simulink model "Appl_HeatFault_CtrlModel"  (R2018b)
settings: configuration reference "CodeConfig_10_ms" (kept outside this file)
undefined symbols (not defined in the file): CAL_CmdOpenTime, CAL_CmdShortTime, CAL_NTCOpenTime, CAL_NTCOverTime, CAL_NTCShortTime, CAL_NTCWaitTime, D_HEATFALUT_CmdOpenLoad, D_HEATFALUT_CmdOpenLoad_W, D_HEATFALUT_CmdShortToGnd, D_HEATFALUT_NtcMax, D_HEATFALUT_NtcMin, D_HEATFALUT_NtcOpenLoad, D_HEATFALUT_NtcShortToGnd, FALSE, TRUE
libraries: DareLib x32, simulink x1
(part 2 of 2)

== stateflow chart Appl_HeatFault_CtrlModel/LogicCtrl/HeatDiagnoseCtrl/HeatDiagnoseDeal/HeatCmdDiagnoseFunction2/HeatCmdDiagnose ==
  state HeatCmdDiagnosis
    state CmdShortToGND
      ex:
      ShortTimer = 0;
      (default) -> (junction 25)
      CmdShortToGND -> (junction 25) [order 1]
      (junction 25) -> (junction 28) [order 1] : /* 未超时 */
          | [CAL_CmdShortTime > ShortTimer]
      (junction 25) -> (junction 30) [order 2] : {ShortTimer = CAL_CmdShortTime;
          | HeatCmdFault = enHeatCmdFault.EN_HEAT_FAULT_GND;
          | HeatCmdFault4DTC = enHeatCmdFault.EN_HEAT_FAULT_GND;}
      (junction 28) -> (junction 32) : {ShortTimer++;}
      (junction 32) -> (junction 30)
      (junction 30) -> (junction 35)
    state ShortLow
    state Default
      en:
      OpenTimer = 0;
      ShortTimer = 0;
      HeatCmdFault =  enHeatCmdFault.EN_HEAT_FAULT_NONE;
      RecoverTimer = 0;
      (default) -> (junction 80)
      Default -> (junction 80) [order 1]
      (junction 80) -> (junction 83) [order 1] : /* 未超时 */
          | [CAL_CmdShortTime > RecoverTimer]
      (junction 80) -> (junction 89) [order 2] : {RecoverTimer = CAL_CmdShortTime;
          | HeatCmdFault4DTC =  enHeatCmdFault.EN_HEAT_FAULT_NONE;}
      (junction 83) -> (junction 84) : {RecoverTimer++;}
      (junction 84) -> (junction 89)
      (junction 89) -> (junction 91)
    state CmdOpenLoad
      ex:
      OpenTimer = 0;
      (default) -> (junction 46)
      CmdOpenLoad -> (junction 46) [order 1]
      (junction 46) -> (junction 43) [order 1] : /* 未超时 */
          | [CAL_CmdOpenTime > OpenTimer]
      (junction 46) -> (junction 47) [order 2] : {OpenTimer = CAL_CmdOpenTime;
          | HeatCmdFault = enHeatCmdFault.EN_HEAT_FAULT_OPEN;
          | HeatCmdFault4DTC = enHeatCmdFault.EN_HEAT_FAULT_OPEN;}
      (junction 43) -> (junction 48) : {OpenTimer++;}
      (junction 48) -> (junction 47)
      (junction 47) -> (junction 40)
    state OpenLow
    CmdShortToGND -> ShortLow [order 1] : /* 低电平 */
        | [enHeatIoSts.EN_HEAT_IO_LOW == HeatIOSts]
    ShortLow -> CmdShortToGND : /* 高电平 */
        | [enHeatIoSts.EN_HEAT_IO_HIGH == HeatIOSts]
    (junction 76) -> CmdShortToGND [order 1] : [FaultType == enHeatCmdFault.EN_HEAT_FAULT_GND]
    Default -> CmdShortToGND [order 1] : /* 输出电流对地短路 */
        | [D_HEATFALUT_CmdShortToGnd < HeatIS]
    CmdShortToGND -> Default [order 2] : /* 输出电流对地短路恢复 */
        | [D_HEATFALUT_CmdShortToGnd >= HeatIS]
    CmdOpenLoad -> CmdShortToGND [order 3] : /* 输出电流对地短路 */
        | [D_HEATFALUT_CmdShortToGnd < HeatIS]
    CmdShortToGND -> CmdOpenLoad [order 3] : /* 输出电流开路 */
        | [D_HEATFALUT_CmdOpenLoad_W > HeatIS]
    (default) -> (junction 76)
    (junction 76) -> Default [order 3]
    (junction 76) -> CmdOpenLoad [order 2] : [FaultType == enHeatCmdFault.EN_HEAT_FAULT_OPEN]
    Default -> CmdOpenLoad [order 2] : /* 输出电流开路 */
        | [D_HEATFALUT_CmdOpenLoad_W > HeatIS]
    CmdOpenLoad -> Default [order 2] : /* 输出电流开路恢复 */
        | [D_HEATFALUT_CmdOpenLoad_W <= HeatIS]
    CmdOpenLoad -> OpenLow [order 1] : /* 低电平 */
        | [enHeatIoSts.EN_HEAT_IO_LOW == HeatIOSts]
    OpenLow -> CmdOpenLoad : /* 高电平 */
        | [enHeatIoSts.EN_HEAT_IO_HIGH == HeatIOSts]
  state HeatCmdClose
    en:
    OpenTimer = 0;
    ShortTimer = 0;
    HeatCmdFault = enHeatCmdFault.EN_HEAT_FAULT_NONE;
    ex:
    HeatCmdFault4DTC = FaultType;
  (default) -> HeatCmdClose
  HeatCmdClose -> HeatCmdDiagnosis : /* 加热CMD */
      | [TRUE == HeatCmd]
  HeatCmdDiagnosis -> HeatCmdClose : /* 无加热CMD */
      | [TRUE != HeatCmd]
  data: HeatIOSts input Enum: enHeatIoSts; HeatCmd input uint8; HeatIS input uint16; HeatCmdFault output Enum: enHeatCmdFault; ShortTimer local uint8; OpenTimer local uint8; CAL_CmdShortTime parameter; CAL_CmdOpenTime parameter; D_HEATFALUT_CmdShortToGnd parameter; D_HEATFALUT_CmdOpenLoad_W parameter; TRUE parameter; HeatCmdFault4DTC output Enum: enHeatCmdFault; FaultType input; RecoverTimer local uint8

== stateflow chart Appl_HeatFault_CtrlModel/LogicCtrl/HeatDiagnoseCtrl/HeatDiagnoseDeal/HeatNTCDiagnoseFunction1/HeatCmdDiagnose ==
  state NTCShortToGND
    ex:
    ShortTimer = 0;
    (default) -> (junction 77)
    NTCShortToGND -> (junction 77) [order 1]
    (junction 77) -> (junction 80) [order 1] : /* 短地超时 */
        | [CAL_NTCShortTime > ShortTimer]
    (junction 77) -> (junction 82) [order 2] : {ShortTimer = CAL_NTCShortTime;
        | HeatNTCFault = enHeatNtcFault.EN_NTC_FAULT_GND;}
    (junction 80) -> (junction 84) : {ShortTimer++;}
    (junction 84) -> (junction 82)
    (junction 82) -> (junction 87)
  state Default
    en:
    WaitAquireTimer = 1;
    RecoveryTimer = 0;
    ex:
    WaitAquireTimer = 0;
    (default) -> (junction 64)
    (junction 64) -> (junction 69) [order 1] : /* 等待超时 */
        | [CAL_NTCWaitTime  > WaitAquireTimer]
    Default -> (junction 64) [order 1]
    (junction 69) -> (junction 71) : {WaitAquireTimer ++;}
    (junction 64) -> (junction 67) [order 2] : {WaitAquireTimer = CAL_NTCWaitTime;}
    (junction 71) -> (junction 67)
    (junction 67) -> (junction 74)
    (junction 74) -> (junction 139) [order 1] : [HeatNTCFault != enHeatNtcFault.EN_NTC_FAULT_NONE]
    (junction 74) -> (junction 162) [order 2]
    (junction 139) -> (junction 141) : {RecoveryTimer++; }
    (junction 141) -> (junction 143) [order 1] : /* NTC不可信故障*/
        | [HeatNTCFault == enHeatNtcFault.EN_NTC_FAULT_UNC]
    (junction 143) -> (junction 145) [order 1] : [/*计时超过5s*/
        | CAL_NTCOverTime < RecoveryTimer]
    (junction 141) -> (junction 152) [order 2]
    (junction 143) -> (junction 158) [order 2]
    (junction 145) -> (junction 150) : {RecoveryTimer = CAL_NTCOverTime;
        | HeatNTCFault = enHeatNtcFault.EN_NTC_FAULT_NONE;}
    (junction 152) -> (junction 154) [order 1] : [/*开路和短地时间皆为1s*/
        | CAL_NTCOpenTime < RecoveryTimer]
    (junction 152) -> (junction 160) [order 2]
    (junction 154) -> (junction 156) : {RecoveryTimer = CAL_NTCOpenTime;
        | HeatNTCFault = enHeatNtcFault.EN_NTC_FAULT_NONE;}
    (junction 162) -> (junction 160)
    (junction 156) -> (junction 160)
    (junction 158) -> (junction 156)
    (junction 150) -> (junction 158)
    (junction 160) -> (junction 168)
  state NTCOpenLoad
    ex:
    OpenTimer = 0;
    (default) -> (junction 94)
    NTCOpenLoad -> (junction 94) [order 1]
    (junction 94) -> (junction 92) [order 1] : /* 开路超时 */
        | [CAL_NTCOpenTime  > OpenTimer]
    (junction 94) -> (junction 95) [order 2] : {OpenTimer = CAL_NTCOpenTime;
        | HeatNTCFault = enHeatNtcFault.EN_NTC_FAULT_OPEN;}
    (junction 92) -> (junction 97) : {OpenTimer ++;}
    (junction 97) -> (junction 95)
    (junction 95) -> (junction 100)
  state NTCOverRange
    ex:
    OverTimer = 0;
    (default) -> (junction 105)
    NTCOverRange -> (junction 105) [order 1]
    (junction 105) -> (junction 108) [order 1] : /* 不可信超时 */
        | [CAL_NTCOverTime   > OverTimer]
    (junction 105) -> (junction 109) [order 2] : {OverTimer = CAL_NTCOverTime ;
        | HeatNTCFault = enHeatNtcFault.EN_NTC_FAULT_UNC;}
    (junction 108) -> (junction 110) : {OverTimer ++;}
    (junction 110) -> (junction 109)
    (junction 109) -> (junction 112)
  NTCShortToGND -> Default [order 1] : /* 对地短路 */
      | [D_HEATFALUT_NtcShortToGnd < HeatNTC]
  Default -> NTCShortToGND [order 1] : /* 对地恢复 */
      | [D_HEATFALUT_NtcShortToGnd >= HeatNTC ...
      | && CAL_NTCWaitTime <= WaitAquireTimer]
  (default) -> Default
  Default -> NTCOpenLoad [order 2] : /* NTC开路 */
      | [D_HEATFALUT_NtcOpenLoad < HeatNTC ...
      | && CAL_NTCWaitTime <= WaitAquireTimer]
  NTCOpenLoad -> Default [order 1] : /* NTC开路恢复*/
      | [D_HEATFALUT_NtcOpenLoad >= HeatNTC]
  Default -> NTCOverRange [order 3] : /* NTC 不可信 */
      | [(NtcMax < HeatNTC ...
      | || NtcMin > HeatNTC) ...
      | && CAL_NTCWaitTime <= WaitAquireTimer]
  NTCOverRange -> Default [order 1] : /* NTC不可信恢复 */
      | [(NtcMax >= HeatNTC && NtcMin <= HeatNTC) ...
      | || D_HEATFALUT_NtcOpenLoad < HeatNTC ...
      | || D_HEATFALUT_NtcShortToGnd >= HeatNTC]
  data: HeatNTC input uint16; HeatNTCFault output Enum: enHeatNtcFault; ShortTimer local uint16; WaitAquireTimer local uint16; OpenTimer local uint16; OverTimer local uint16; CAL_NTCOpenTime parameter; CAL_NTCOverTime parameter; CAL_NTCShortTime parameter; CAL_NTCWaitTime parameter; D_HEATFALUT_NtcOpenLoad parameter; D_HEATFALUT_NtcShortToGnd parameter; RecoveryTimer local uint16; NtcMin input uint16; NtcMax input uint16

== stateflow chart Appl_HeatFault_CtrlModel/LogicCtrl/HeatDiagnoseCtrl/HeatDiagnoseDeal/HeatNTCDiagnoseFunction2/HeatCmdDiagnose ==
  state NTCShortToGND
    ex:
    ShortTimer = 0;
    (default) -> (junction 77)
    NTCShortToGND -> (junction 77) [order 1]
    (junction 77) -> (junction 80) [order 1] : /* 短地超时 */
        | [CAL_NTCShortTime > ShortTimer]
    (junction 77) -> (junction 82) [order 2] : {ShortTimer = CAL_NTCShortTime;
        | HeatNTCFault = enHeatNtcFault.EN_NTC_FAULT_GND;}
    (junction 80) -> (junction 84) : {ShortTimer++;}
    (junction 84) -> (junction 82)
    (junction 82) -> (junction 87)
  state Default
    en:
    WaitAquireTimer = 1;
    RecoveryTimer = 0;
    ex:
    WaitAquireTimer = 0;
    (default) -> (junction 64)
    (junction 64) -> (junction 69) [order 1] : /* 等待超时 */
        | [CAL_NTCWaitTime  > WaitAquireTimer]
    Default -> (junction 64) [order 1]
    (junction 69) -> (junction 71) : {WaitAquireTimer ++;}
    (junction 64) -> (junction 67) [order 2] : {WaitAquireTimer = CAL_NTCWaitTime;}
    (junction 71) -> (junction 67)
    (junction 67) -> (junction 74)
    (junction 74) -> (junction 139) [order 1] : [HeatNTCFault != enHeatNtcFault.EN_NTC_FAULT_NONE]
    (junction 74) -> (junction 162) [order 2]
    (junction 139) -> (junction 141) : {RecoveryTimer++; }
    (junction 141) -> (junction 143) [order 1] : /* NTC不可信故障*/
        | [HeatNTCFault == enHeatNtcFault.EN_NTC_FAULT_UNC]
    (junction 143) -> (junction 145) [order 1] : [/*计时超过5s*/
        | CAL_NTCOverTime < RecoveryTimer]
    (junction 141) -> (junction 152) [order 2]
    (junction 143) -> (junction 158) [order 2]
    (junction 145) -> (junction 150) : {RecoveryTimer = CAL_NTCOverTime;
        | HeatNTCFault = enHeatNtcFault.EN_NTC_FAULT_NONE;}
    (junction 152) -> (junction 154) [order 1] : [/*开路和短地时间皆为1s*/
        | CAL_NTCOpenTime < RecoveryTimer]
    (junction 152) -> (junction 160) [order 2]
    (junction 154) -> (junction 156) : {RecoveryTimer = CAL_NTCOpenTime;
        | HeatNTCFault = enHeatNtcFault.EN_NTC_FAULT_NONE;}
    (junction 162) -> (junction 160)
    (junction 156) -> (junction 160)
    (junction 158) -> (junction 156)
    (junction 150) -> (junction 158)
    (junction 160) -> (junction 168)
  state NTCOpenLoad
    ex:
    OpenTimer = 0;
    (default) -> (junction 94)
    NTCOpenLoad -> (junction 94) [order 1]
    (junction 94) -> (junction 92) [order 1] : /* 开路超时 */
        | [CAL_NTCOpenTime  > OpenTimer]
    (junction 94) -> (junction 95) [order 2] : {OpenTimer = CAL_NTCOpenTime;
        | HeatNTCFault = enHeatNtcFault.EN_NTC_FAULT_OPEN;}
    (junction 92) -> (junction 97) : {OpenTimer ++;}
    (junction 97) -> (junction 95)
    (junction 95) -> (junction 100)
  state NTCOverRange
    ex:
    OverTimer = 0;
    (default) -> (junction 105)
    NTCOverRange -> (junction 105) [order 1]
    (junction 105) -> (junction 108) [order 1] : /* 不可信超时 */
        | [CAL_NTCOverTime   > OverTimer]
    (junction 105) -> (junction 109) [order 2] : {OverTimer = CAL_NTCOverTime ;
        | HeatNTCFault = enHeatNtcFault.EN_NTC_FAULT_UNC;}
    (junction 108) -> (junction 110) : {OverTimer ++;}
    (junction 110) -> (junction 109)
    (junction 109) -> (junction 112)
  NTCShortToGND -> Default [order 1] : /* 对地短路 */
      | [D_HEATFALUT_NtcShortToGnd < HeatNTC]
  Default -> NTCShortToGND [order 1] : /* 对地恢复 */
      | [D_HEATFALUT_NtcShortToGnd >= HeatNTC ...
      | && CAL_NTCWaitTime <= WaitAquireTimer]
  (default) -> Default
  Default -> NTCOpenLoad [order 2] : /* NTC开路 */
      | [D_HEATFALUT_NtcOpenLoad < HeatNTC ...
      | && CAL_NTCWaitTime <= WaitAquireTimer]
  NTCOpenLoad -> Default [order 1] : /* NTC开路恢复*/
      | [D_HEATFALUT_NtcOpenLoad >= HeatNTC]
  Default -> NTCOverRange [order 3] : /* NTC 不可信 */
      | [(NtcMax < HeatNTC ...
      | || NtcMin > HeatNTC) ...
      | && CAL_NTCWaitTime <= WaitAquireTimer]
  NTCOverRange -> Default [order 1] : /* NTC不可信恢复 */
      | [(NtcMax >= HeatNTC && NtcMin <= HeatNTC) ...
      | || D_HEATFALUT_NtcOpenLoad < HeatNTC ...
      | || D_HEATFALUT_NtcShortToGnd >= HeatNTC]
  data: HeatNTC input uint16; HeatNTCFault output Enum: enHeatNtcFault; ShortTimer local uint16; WaitAquireTimer local uint16; OpenTimer local uint16; OverTimer local uint16; CAL_NTCOpenTime parameter; CAL_NTCOverTime parameter; CAL_NTCShortTime parameter; CAL_NTCWaitTime parameter; D_HEATFALUT_NtcOpenLoad parameter; D_HEATFALUT_NtcShortToGnd parameter; RecoveryTimer local uint16; NtcMin input uint16; NtcMax input uint16

== stateflow chart Appl_HeatFault_CtrlModel/UpDataInputInfo/InputSignalProcess/CMD_Process/GetFaultType ==
  state FaultType = getFaultType(ShortGND,Openload) [function]
  state GetFaultType
    du:
    DrFaultType = getFaultType(HeatFalut_DrCmdShortGND,HeatFalut_DrCmdOpenload);
    PaFaultType = getFaultType(HeatFalut_PaCmdShortGND,HeatFalut_PaCmdOpenload);
    ThirdFaultType = getFaultType(HeatFalut_3rdCmdShortGND,HeatFalut_3rdCmdOpenload);
  (default) -> GetFaultType
  data: FaultType function_output; ShortGND function_input; Openload function_input; HeatFalut_DrCmdShortGND input; HeatFalut_PaCmdShortGND input; EN_HEAT_FAULT_GND local double; EN_HEAT_FAULT_NONE local double; EN_HEAT_FAULT_OPEN local double; TRUE local double; HeatFalut_3rdCmdShortGND input; HeatFalut_DrCmdOpenload input; HeatFalut_PaCmdOpenload input; HeatFalut_3rdCmdOpenload input; DrFaultType output Enum: enHeatCmdFault; PaFaultType output Enum: enHeatCmdFault; ThirdFaultType output Enum: enHeatCmdFault

== stateflow chart Appl_HeatFault_CtrlModel/UpDataInputInfo/InputSignalProcess/CMD_Process/GetFaultType/getFaultType/Chart ==
  (default) -> (junction 1)
  (junction 1) -> (junction 9) [order 2] : [TRUE == Openload]
  (junction 1) -> (junction 3) [order 1] : [TRUE == ShortGND]
  (junction 9) -> (junction 11) : {FaultType = enHeatCmdFault.EN_HEAT_FAULT_OPEN}
  (junction 1) -> (junction 7) [order 3] : {FaultType = enHeatCmdFault.EN_HEAT_FAULT_NONE;}
  (junction 3) -> (junction 5) : {FaultType = enHeatCmdFault.EN_HEAT_FAULT_GND;}
  (junction 11) -> (junction 7)
  (junction 5) -> (junction 7)
  (junction 7) -> (junction 15)
  data: ShortGND input uint8; Openload input uint8; FaultType output uint8; TRUE parameter
